simulink model "q_heli_2d_ff_lqr_i_no_joystick"  (Simulink 8.8)
settings: Solver=FixedStepAuto  StartTime=0.0  StopTime=inf  FixedStep=1e-3  MaxStep=10  RelTol=1e-3  AbsTol=1e-3
values from neighbouring files (symbols this model uses):
  B_p = 0.3    [parametri.m]
  B_y = 0.45    [parametri.m]
  g = 9.81    [parametri.m]    (also in setup_heli_2d_configuration.m)
  J_eq_p = J_p - m_heli*l_cm^2    (= 0.014688525)    [parametri.m]    (also in setup_heli_2d_configuration.m = 0.0181734333333)
  J_eq_y = J_y - m_heli*l_cm^2    (= 0.016488525)    [parametri.m]    (also in setup_heli_2d_configuration.m = 0.02311385)
  K_AMP = 1    [setup_lab_heli_2d.m]
  K_EC_P = 2 * pi / 2400    (= 0.00261799387799)    [setup_lab_heli_2d.m]
  K_EC_Y = 2 * pi / 2400    (= 0.00261799387799)    [setup_lab_heli_2d.m]
  K_ff = 1    [setup_lab_heli_2d.m]
  K_pp = 0.35 * d_p    (= 0.06825)    [parametri.m]    (also in setup_heli_2d_configuration.m = 0.18)
  K_py = 0.018    [parametri.m]    (also in setup_heli_2d_configuration.m = 0.06875)
  K_yp = 0.018    [parametri.m]    (also in setup_heli_2d_configuration.m = 0.06875)
  K_yy = 0.35 * d_y    (= 0.06475)    [parametri.m]    (also in setup_heli_2d_configuration.m = 0.162)
  l_cm = 0.005    [parametri.m]    (also in setup_heli_2d_configuration.m = 0.19)
  m_heli = 2*(m_propeler + m_motor + m_motor_drzac) + m_sipka + m_drzac    (= 0.459)    [parametri.m]    (also in setup_heli_2d_configuration.m = 0.6)
  SAT_INT_ERR_PITCH = 3.2    [setup_lab_heli_2d.m]
  SAT_INT_ERR_YAW = 3.2    [setup_lab_heli_2d.m]
  theta_0 = -47*pi/180    (= -0.820304748437)    [setup_lab_heli_2d.m]
  Tr_p = 1    [setup_lab_heli_2d.m]
  Tr_y = 1    [setup_lab_heli_2d.m]
  VMAX_AMP_P = 3.2    [setup_lab_heli_2d.m]
  VMAX_AMP_Y = 3.2    [setup_lab_heli_2d.m]
  wcf = 2 * pi * 20    (= 125.663706144)    [setup_lab_heli_2d.m]
  zetaf = 0.85    [setup_lab_heli_2d.m]
undefined symbols (not defined in the file or in its folder): K, Ki, MultiQ, PCI, Quanser
libraries: simulink x9, simulink_extras x5, sldrtlib x4
settings Model: Creator=MLevis  LastModifiedBy=Labos1  SimulationMode=external  ExtModeTrigDuration=50000
settings SolverCC: PositivePriorityOrder=on
settings DataIOCC: LimitDataPoints=off  SaveOutput=off  SaveTime=off  SignalLoggingName=sigsOut
settings OptimizationCC: BlockReduction=off  BooleanDataType=off  OptimizeBlockIOStorage=off  BufferReuse=off  GlobalBufferReuse=off  ExpressionFolding=off  ExpressionDepthLimit=2147483647  LocalBlockOutputs=off  InitFltsAndDblsToZero=on  LifeSpan=auto
settings DebuggingCC: SaveWithParameterizedLinksMsg=none  SignalResolutionControl=TryResolveAllWithWarning  MultiTaskDSMMsg=warning  MultiTaskCondExecSysMsg=none
settings HardwareCC: ProdBitPerPointer=64  ProdBitPerSizeT=64  ProdBitPerPtrDiffT=64  ProdLargestAtomicFloat=Float  ProdIntDivRoundTo=Zero  ProdEndianess=LittleEndian  ProdWordSize=64  ProdHWDeviceType=Intel->x86-64 (Windows64)
settings RTWCC: SystemTargetFile=sldrt.tlc  TemplateMakefile=sldrt.tmf  Description=Simulink Desktop Real-Time  RTWCompilerOptimization=on
settings CodeAppCC: MaxIdLength=95
settings SimulinkDesktopRealTimeCC: TargetPreCompLibLocation=C:\Program Files\MATLAB\R2016b\toolbox\sldrt\lib\win64  TargetLangStandard=C89/C90 (ANSI)  SupportVariableSizeSignals=off

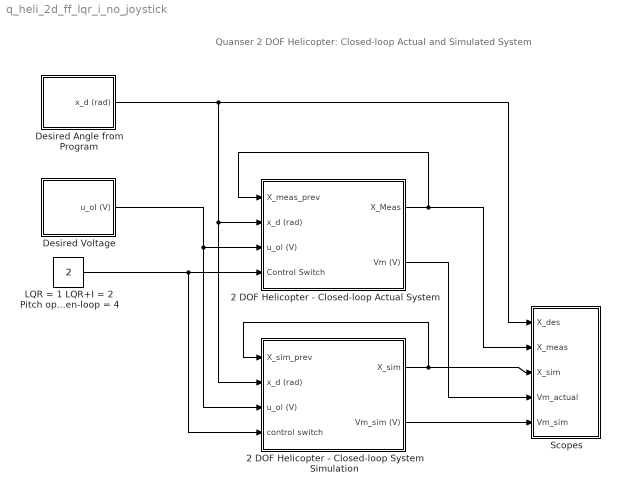
== system q_heli_2d_ff_lqr_i_no_joystick ==
  note: Quanser 2 DOF Helicopter:
      | Closed-loop Actual and Simulated System
  2 DOF Helicopter - Closed-loop Actual System : Subsystem
  2 DOF Helicopter - Closed-loop System Simulation : Subsystem
  Desired Angle from Program : Subsystem
  Desired Voltage : Subsystem
  LQR = 1 LQR+I = 2 Pitch open-loop  = 3 Yaw open-loop = 4 : Constant  Value=2
  Scopes : Subsystem
  wires:
  2 DOF Helicopter - Closed-loop System Simulation/1(X_sim) -> Scopes/3(X_sim), 2 DOF Helicopter - Closed-loop System Simulation/1(X_sim_prev)
  2 DOF Helicopter - Closed-loop Actual System/1(X_Meas) -> 2 DOF Helicopter - Closed-loop Actual System/1(X_meas_prev), Scopes/2(X_meas)
  2 DOF Helicopter - Closed-loop Actual System/2(Vm (V)) -> Scopes/4(Vm_actual)
  LQR = 1 LQR+I = 2 Pitch open-loop  = 3 Yaw open-loop = 4/1 -> 2 DOF Helicopter - Closed-loop Actual System/4(Control Switch), 2 DOF Helicopter - Closed-loop System Simulation/4(control switch)
  2 DOF Helicopter - Closed-loop System Simulation/2(Vm_sim (V)) -> Scopes/5(Vm_sim)
  Desired Voltage/1(u_ol (V)) -> 2 DOF Helicopter - Closed-loop Actual System/3(u_ol (V)), 2 DOF Helicopter - Closed-loop System Simulation/3(u_ol (V))
  Desired Angle from Program/1(x_d (rad)) -> Scopes/1(X_des), 2 DOF Helicopter - Closed-loop Actual System/2(x_d (rad)), 2 DOF Helicopter - Closed-loop System Simulation/2(x_d (rad))

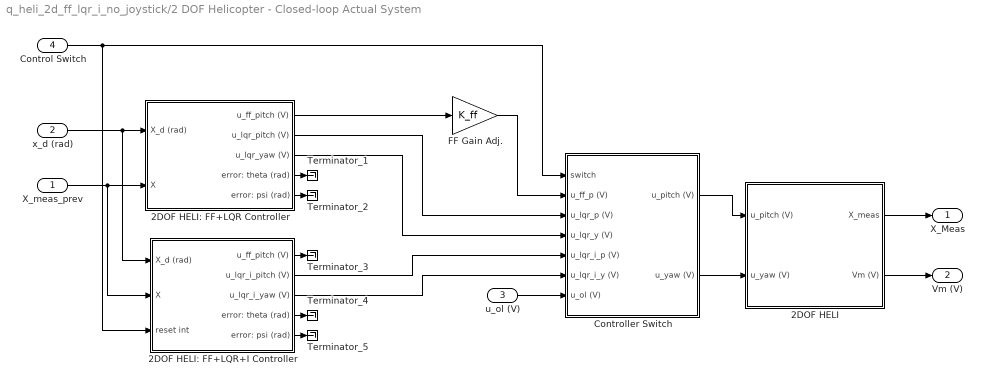
== system q_heli_2d_ff_lqr_i_no_joystick/2 DOF Helicopter - Closed-loop Actual System ==
  X_meas_prev : Inport
  x_d (rad) : Inport  Port=2
  u_ol (V) : Inport  Port=3
  Control Switch : Inport  Port=4
  2DOF HELI : Subsystem
  2DOF HELI: FF+LQR Controller : Subsystem
  2DOF HELI: FF+LQR+I Controller : Subsystem
  Controller Switch : Subsystem
  FF Gain Adj. : Gain  Gain=K_ff
  Terminator_{1..5} (5 alike) : Terminator
  X_Meas : Outport
  Vm (V) : Outport  Port=2
  wires:
  2DOF HELI/1(X_meas) -> X_Meas/1
  2DOF HELI/2(Vm (V)) -> Vm (V)/1
  Control Switch/1 -> 2DOF HELI: FF+LQR+I Controller/3(reset int), Controller Switch/1(switch)
  2DOF HELI: FF+LQR Controller/1(u_ff_pitch (V)) -> FF Gain Adj./1
  x_d (rad)/1 -> 2DOF HELI: FF+LQR Controller/1(X_d (rad)), 2DOF HELI: FF+LQR+I Controller/1(X_d (rad))
  X_meas_prev/1 -> 2DOF HELI: FF+LQR Controller/2(X), 2DOF HELI: FF+LQR+I Controller/2(X)
  2DOF HELI: FF+LQR Controller/3(u_lqr_yaw (V)) -> Controller Switch/4(u_lqr_y (V))
  FF Gain Adj./1 -> Controller Switch/2(u_ff_p (V))
  2DOF HELI: FF+LQR Controller/2(u_lqr_pitch (V)) -> Controller Switch/3(u_lqr_p (V))
  Controller Switch/1(u_pitch (V)) -> 2DOF HELI/1(u_pitch (V))
  Controller Switch/2(u_yaw (V)) -> 2DOF HELI/2(u_yaw (V))
  2DOF HELI: FF+LQR+I Controller/2(u_lqr_i_pitch (V)) -> Controller Switch/5(u_lqr_i_p (V))
  2DOF HELI: FF+LQR+I Controller/3(u_lqr_i_yaw (V)) -> Controller Switch/6(u_lqr_i_y (V))
  u_ol (V)/1 -> Controller Switch/7(u_ol (V))
  2DOF HELI: FF+LQR Controller/4(error: theta (rad)) -> Terminator_1/1
  2DOF HELI: FF+LQR Controller/5(error: psi (rad)) -> Terminator_2/1
  2DOF HELI: FF+LQR+I Controller/1(u_ff_pitch (V)) -> Terminator_3/1
  2DOF HELI: FF+LQR+I Controller/4(error: theta (rad)) -> Terminator_4/1
  2DOF HELI: FF+LQR+I Controller/5(error: psi (rad)) -> Terminator_5/1

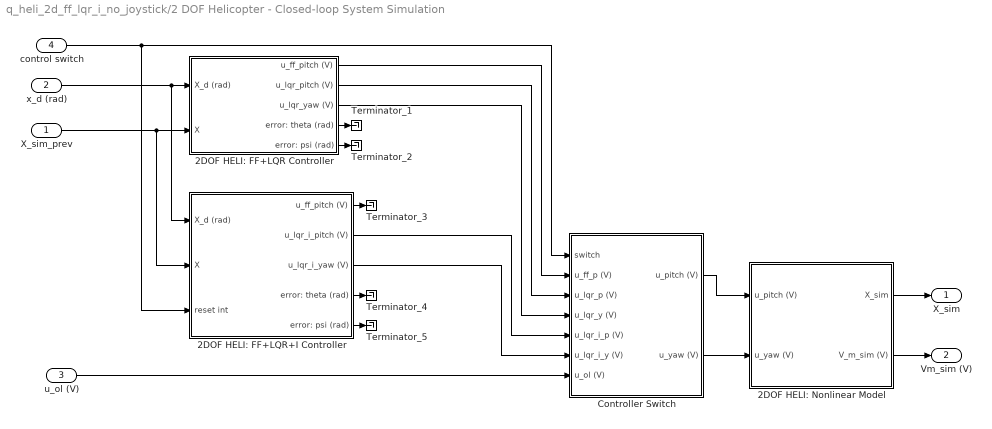
== system q_heli_2d_ff_lqr_i_no_joystick/2 DOF Helicopter - Closed-loop System Simulation ==
  X_sim_prev : Inport
  x_d (rad) : Inport  Port=2
  u_ol (V) : Inport  Port=3
  control switch : Inport  Port=4
  2DOF HELI: FF+LQR Controller : Subsystem
  2DOF HELI: FF+LQR+I Controller : Subsystem
  2DOF HELI: Nonlinear Model : Subsystem
  Controller Switch : Subsystem
  Terminator_{1..5} (5 alike) : Terminator
  X_sim : Outport
  Vm_sim (V) : Outport  Port=2
  wires:
  Controller Switch/2(u_yaw (V)) -> 2DOF HELI: Nonlinear Model/2(u_yaw (V))
  Controller Switch/1(u_pitch (V)) -> 2DOF HELI: Nonlinear Model/1(u_pitch (V))
  x_d (rad)/1 -> 2DOF HELI: FF+LQR+I Controller/1(X_d (rad)), 2DOF HELI: FF+LQR Controller/1(X_d (rad))
  X_sim_prev/1 -> 2DOF HELI: FF+LQR Controller/2(X), 2DOF HELI: FF+LQR+I Controller/2(X)
  2DOF HELI: FF+LQR+I Controller/3(u_lqr_i_yaw (V)) -> Controller Switch/6(u_lqr_i_y (V))
  2DOF HELI: FF+LQR Controller/2(u_lqr_pitch (V)) -> Controller Switch/3(u_lqr_p (V))
  2DOF HELI: FF+LQR Controller/1(u_ff_pitch (V)) -> Controller Switch/2(u_ff_p (V))
  2DOF HELI: FF+LQR Controller/3(u_lqr_yaw (V)) -> Controller Switch/4(u_lqr_y (V))
  2DOF HELI: FF+LQR+I Controller/2(u_lqr_i_pitch (V)) -> Controller Switch/5(u_lqr_i_p (V))
  control switch/1 -> Controller Switch/1(switch), 2DOF HELI: FF+LQR+I Controller/3(reset int)
  2DOF HELI: Nonlinear Model/2(V_m_sim (V)) -> Vm_sim (V)/1
  2DOF HELI: Nonlinear Model/1(X_sim) -> X_sim/1
  u_ol (V)/1 -> Controller Switch/7(u_ol (V))
  2DOF HELI: FF+LQR Controller/4(error: theta (rad)) -> Terminator_1/1
  2DOF HELI: FF+LQR Controller/5(error: psi (rad)) -> Terminator_2/1
  2DOF HELI: FF+LQR+I Controller/1(u_ff_pitch (V)) -> Terminator_3/1
  2DOF HELI: FF+LQR+I Controller/4(error: theta (rad)) -> Terminator_4/1
  2DOF HELI: FF+LQR+I Controller/5(error: psi (rad)) -> Terminator_5/1

== system q_heli_2d_ff_lqr_i_no_joystick/Desired Angle from Program ==
  note: Desired pitch angle
  note: Desired yaw angle
  Amplitude: Pitch (deg) : Gain
  Amplitude: Yaw (deg) : Gain
  Constant : Constant
  Constant: Pitch (deg) : simulink/Math Operations/Slider Gain  low=-50  gain=0  high=25
  Constant: Yaw (deg) : Constant  Value=0
  Mux : Mux  Inputs=2
  Pitch: deg to rad : simulink_extras/Transformations/Degrees to Radians
  Signal Generator: Pitch : SignalGenerator  WaveForm=square  Amplitude=20  Frequency=0.05
  Signal Generator: Yaw : SignalGenerator  WaveForm=square  Amplitude=45  Frequency=0.05
  Sum : Sum  Inputs=|++
  Sum1 : Sum  Inputs=|++
  Yaw: deg to rad : simulink_extras/Transformations/Degrees to Radians
  x_d (rad) : Outport
  wires:
  Pitch: deg to rad/1 -> Mux/1
  Sum/1 -> Pitch: deg to rad/1
  Signal Generator: Pitch/1 -> Amplitude: Pitch (deg)/1
  Amplitude: Pitch (deg)/1 -> Sum/1
  Constant/1 -> Constant: Pitch (deg)/1
  Sum1/1 -> Yaw: deg to rad/1
  Signal Generator: Yaw/1 -> Amplitude: Yaw (deg)/1
  Amplitude: Yaw (deg)/1 -> Sum1/1
  Constant: Yaw (deg)/1 -> Sum1/2
  Mux/1 -> x_d (rad)/1
  Yaw: deg to rad/1 -> Mux/2
  Constant: Pitch (deg)/1 -> Sum/2

== system q_heli_2d_ff_lqr_i_no_joystick/Desired Voltage ==
  note: Desired pitch open-loop voltage
  note: Desired yaw open-loop voltage
  Amplitude: Pitch (V) : Gain  Gain=0
  Amplitude: Yaw (V) : Gain  Gain=0
  Constant: Pitch (V) : Constant  Value=0
  Constant: Yaw (V) : Constant  Value=0
  Mux : Mux  Inputs=2
  Signal Generator: Pitch (V) : SignalGenerator  WaveForm=square  Frequency=0.4
  Signal Generator: Yaw (V) : SignalGenerator  WaveForm=square  Frequency=0.01
  Sum : Sum  Inputs=|++
  Sum1 : Sum  Inputs=|++
  u_ol (V) : Outport
  wires:
  Constant: Pitch (V)/1 -> Sum/2
  Amplitude: Pitch (V)/1 -> Sum/1
  Signal Generator: Pitch (V)/1 -> Amplitude: Pitch (V)/1
  Constant: Yaw (V)/1 -> Sum1/2
  Amplitude: Yaw (V)/1 -> Sum1/1
  Signal Generator: Yaw (V)/1 -> Amplitude: Yaw (V)/1
  Sum/1 -> Mux/1
  Sum1/1 -> Mux/2
  Mux/1 -> u_ol (V)/1

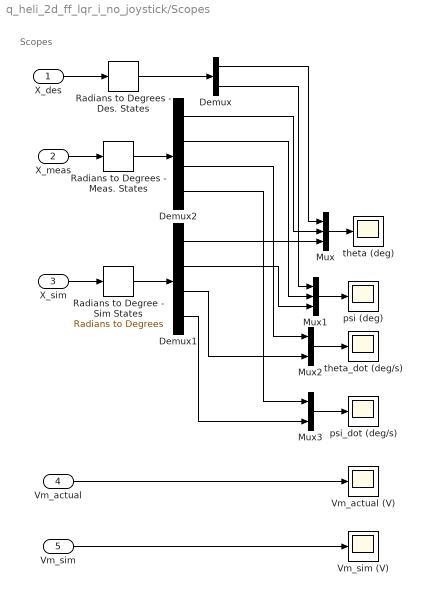
== system q_heli_2d_ff_lqr_i_no_joystick/Scopes ==
  note: Scopes
  X_des : Inport
  X_meas : Inport  Port=2
  X_sim : Inport  Port=3
  Vm_actual : Inport  Port=4
  Vm_sim : Inport  Port=5
  Demux : Demux  Outputs=2
  Demux1 : Demux
  Demux2 : Demux
  Mux : Mux  Inputs=3
  Mux1 : Mux  Inputs=3
  Mux2 : Mux  Inputs=2
  Mux3 : Mux  Inputs=2
  Radians to Degree - Sim States : simulink_extras/Transformations/Radians to Degrees
  Radians to Degrees - Des. States : simulink_extras/Transformations/Radians to Degrees
  Radians to Degrees - Meas. States : simulink_extras/Transformations/Radians to Degrees
  Vm_actual (V) : Scope
  Vm_sim (V) : Scope
  psi (deg) : Scope
  psi_dot (deg/s) : Scope
  theta (deg) : Scope
  theta_dot (deg/s) : Scope
  wires:
  Vm_sim/1 -> Vm_sim (V)/1
  Radians to Degrees - Des. States/1 -> Demux/1
  Demux1/2 -> Mux1/3
  Demux2/2 -> Mux1/2
  Demux/2 -> Mux1/1
  Demux1/1 -> Mux/3
  Demux2/1 -> Mux/2
  Demux/1 -> Mux/1
  X_des/1 -> Radians to Degrees - Des. States/1
  Demux2/3 -> Mux2/1
  Demux2/4 -> Mux3/1
  X_meas/1 -> Radians to Degrees - Meas. States/1
  Radians to Degrees - Meas. States/1 -> Demux2/1
  X_sim/1 -> Radians to Degree - Sim States/1
  Radians to Degree - Sim States/1 -> Demux1/1
  Mux/1 -> theta (deg)/1
  Mux1/1 -> psi (deg)/1
  Mux2/1 -> theta_dot (deg/s)/1
  Mux3/1 -> psi_dot (deg/s)/1
  Demux1/3 -> Mux2/2
  Demux1/4 -> Mux3/2
  Vm_actual/1 -> Vm_actual (V)/1

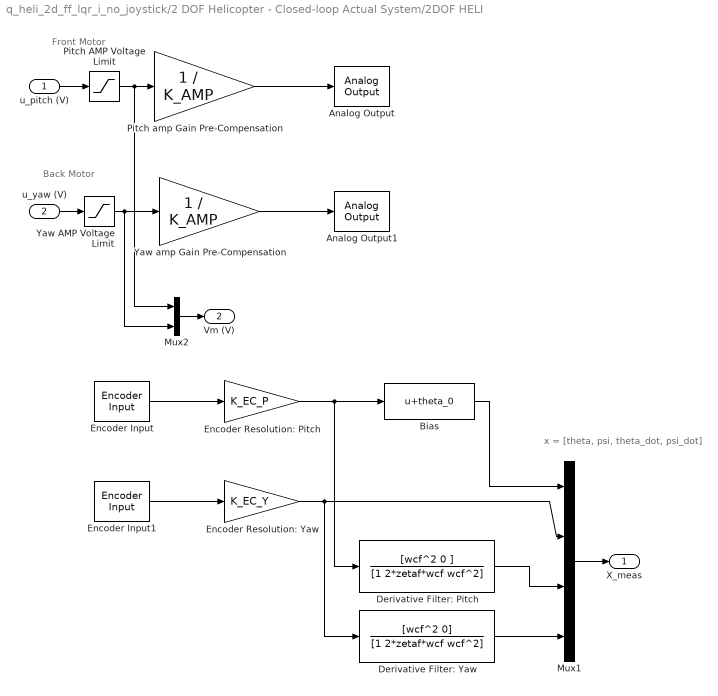
== system q_heli_2d_ff_lqr_i_no_joystick/2 DOF Helicopter - Closed-loop Actual System/2DOF HELI ==
  note: Back Motor
  note: Front Motor
  note: x = [theta, psi, theta_dot, psi_dot]
  u_pitch (V) : Inport
  u_yaw (V) : Inport  Port=2
  Analog Output : sldrtlib/Analog Output  SampleTime=1e-3  MaxMissedTicks=10  ShowMissedTicks=off  YieldWhenWaiting=off  DrvName=Quanser/MultiQ-PCI  DrvAddress=4294967295  DrvOptions=zeros(1,0)  Channels=1  RangeMode=1  VoltRange=1  InitialValue=0  FinalValue=0
      settings: AttributesFormatString=Quanser\nMultiQ-PCI [auto]
  Analog Output1 : sldrtlib/Analog Output  SampleTime=1e-3  MaxMissedTicks=10  ShowMissedTicks=off  YieldWhenWaiting=off  DrvName=Quanser/MultiQ-PCI  DrvAddress=4294967295  DrvOptions=zeros(1,0)  Channels=2  RangeMode=1  VoltRange=1  InitialValue=0  FinalValue=0
      settings: AttributesFormatString=Quanser\nMultiQ-PCI [auto]
  Bias : Bias  Bias=theta_0
  Derivative Filter: Pitch : TransferFcn  Numerator=[wcf^2 0 ]  Denominator=[1 2*zetaf*wcf wcf^2]
  Derivative Filter: Yaw : TransferFcn  Numerator=[wcf^2 0]  Denominator=[1 2*zetaf*wcf wcf^2]
  Encoder Input : sldrtlib/Encoder Input  SampleTime=1e-3  MaxMissedTicks=10  ShowMissedTicks=off  YieldWhenWaiting=off  DrvName=Quanser/MultiQ-PCI  DrvAddress=4294967295  DrvOptions=zeros(1,0)  Channels=1  QuadMode=3  IndexPulse=2  InputFilter=Inf  DataType=1
      settings: AttributesFormatString=Quanser\nMultiQ-PCI [auto]
  Encoder Input1 : sldrtlib/Encoder Input  SampleTime=1e-3  MaxMissedTicks=10  ShowMissedTicks=off  YieldWhenWaiting=off  DrvName=Quanser/MultiQ-PCI  DrvAddress=4294967295  DrvOptions=zeros(1,0)  Channels=2  QuadMode=3  IndexPulse=2  InputFilter=Inf  DataType=1
      settings: AttributesFormatString=Quanser\nMultiQ-PCI [auto]
  "Encoder Resolution: Pitch " : Gain  Gain=K_EC_P
  Encoder Resolution: Yaw : Gain  Gain=K_EC_Y
  Mux1 : Mux
  Mux2 : Mux  Inputs=2
  Pitch AMP Voltage Limit : Saturate  UpperLimit=VMAX_AMP_P  LowerLimit=- VMAX_AMP_P
  Pitch amp Gain Pre-Compensation : Gain  Gain=1 / K_AMP  SaturateOnIntegerOverflow=on  OutDataTypeStr=Inherit: Same as input  ParamDataTypeStr=Inherit: Same as input
  Yaw AMP Voltage Limit : Saturate  UpperLimit=VMAX_AMP_Y  LowerLimit=- VMAX_AMP_Y
  Yaw amp Gain Pre-Compensation : Gain  Gain=1 / K_AMP  SaturateOnIntegerOverflow=on  OutDataTypeStr=Inherit: Same as input  ParamDataTypeStr=Inherit: Same as input
  X_meas : Outport
  Vm (V) : Outport  Port=2
  wires:
  Encoder Resolution: Yaw/1 -> Mux1/2, Derivative Filter: Yaw/1
  Mux2/1 -> Vm (V)/1
  Mux1/1 -> X_meas/1
  u_yaw (V)/1 -> Yaw AMP Voltage Limit/1
  u_pitch (V)/1 -> Pitch AMP Voltage Limit/1
  Yaw AMP Voltage Limit/1 -> Mux2/2, Yaw amp Gain Pre-Compensation/1
  Pitch AMP Voltage Limit/1 -> Mux2/1, Pitch amp Gain Pre-Compensation/1
  Encoder Input/1 -> "Encoder Resolution: Pitch "/1
  "Encoder Resolution: Pitch "/1 -> Bias/1, Derivative Filter: Pitch/1
  Bias/1 -> Mux1/1
  Derivative Filter: Pitch/1 -> Mux1/3
  Derivative Filter: Yaw/1 -> Mux1/4
  Pitch amp Gain Pre-Compensation/1 -> Analog Output/1
  Yaw amp Gain Pre-Compensation/1 -> Analog Output1/1
  Encoder Input1/1 -> Encoder Resolution: Yaw/1

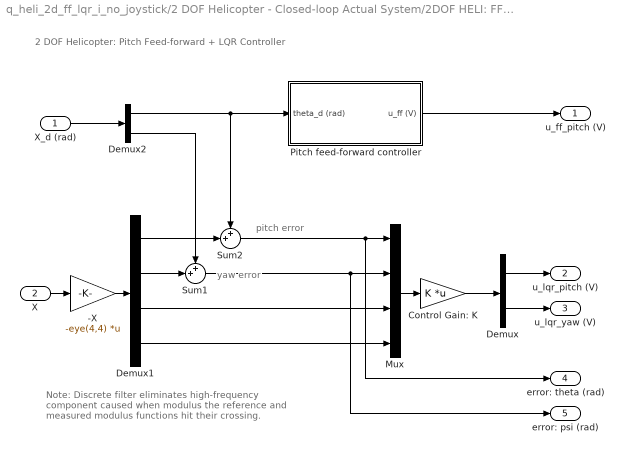
== system q_heli_2d_ff_lqr_i_no_joystick/2 DOF Helicopter - Closed-loop Actual System/2DOF HELI: FF+LQR Controller ==
  note: Note: Discrete filter eliminates high-frequency
      | component caused when modulus the reference
      | and measured modulus functions hit their crossing.
  note: 2 DOF Helicopter:
      | Pitch Feed-forward + LQR Controller
  note: pitch error
  note: yaw error
  X_d (rad) : Inport
  X : Inport  Port=2
  -X : Gain  Gain=-eye(4,4)  Multiplication=Matrix(K*u)
  Control Gain: K : Gain  Gain=K  Multiplication=Matrix(K*u)
  Demux : Demux  Outputs=2
  Demux1 : Demux
  Demux2 : Demux  Outputs=2
  Mux : Mux
  Pitch feed-forward controller : Subsystem
  Sum1 : Sum  Inputs=++|
  Sum2 : Sum  Inputs=++|
  u_ff_pitch (V) : Outport
  u_lqr_pitch (V) : Outport  Port=2
  u_lqr_yaw (V) : Outport  Port=3
  error: theta (rad) : Outport  Port=4
  error: psi (rad) : Outport  Port=5
  wires:
  Sum1/1 -> error: psi (rad)/1, Mux/2
  Demux2/1 -> Sum2/1, Pitch feed-forward controller/1(theta_d (rad))
  Demux2/2 -> Sum1/1
  Demux1/2 -> Sum1/2
  X_d (rad)/1 -> Demux2/1
  Demux1/4 -> Mux/4
  Demux1/3 -> Mux/3
  Mux/1 -> Control Gain: K/1
  Control Gain: K/1 -> Demux/1
  -X/1 -> Demux1/1
  X/1 -> -X/1
  Demux1/1 -> Sum2/2
  Sum2/1 -> error: theta (rad)/1, Mux/1
  Demux/2 -> u_lqr_yaw (V)/1
  Demux/1 -> u_lqr_pitch (V)/1
  Pitch feed-forward controller/1(u_ff (V)) -> u_ff_pitch (V)/1

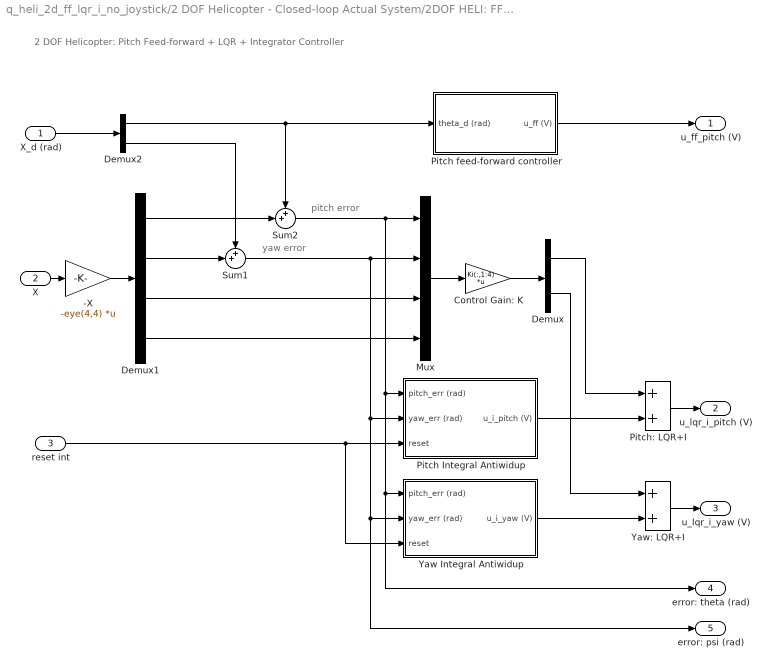
== system q_heli_2d_ff_lqr_i_no_joystick/2 DOF Helicopter - Closed-loop Actual System/2DOF HELI: FF+LQR+I Controller ==
  note: yaw error
  note: pitch error
  note: 2 DOF Helicopter:
      | Pitch Feed-forward + LQR + Integrator Controller
  X_d (rad) : Inport
  X : Inport  Port=2
  reset int : Inport  Port=3
  -X : Gain  Gain=-eye(4,4)  Multiplication=Matrix(K*u)
  Control Gain: K : Gain  Gain=Ki(:,1:4)  Multiplication=Matrix(K*u)
  Demux : Demux  Outputs=2
  Demux1 : Demux
  Demux2 : Demux  Outputs=2
  Mux : Mux
  Pitch Integral Antiwidup : Subsystem
  Pitch feed-forward controller : Subsystem
  Pitch: LQR+I : Sum
  Sum1 : Sum  Inputs=++|
  Sum2 : Sum  Inputs=++|
  Yaw Integral Antiwidup : Subsystem
  Yaw: LQR+I : Sum
  u_ff_pitch (V) : Outport
  u_lqr_i_pitch (V) : Outport  Port=2
  u_lqr_i_yaw (V) : Outport  Port=3
  error: theta (rad) : Outport  Port=4
  error: psi (rad) : Outport  Port=5
  wires:
  reset int/1 -> Pitch Integral Antiwidup/3(reset), Yaw Integral Antiwidup/3(reset)
  Demux1/2 -> Sum1/2
  Demux2/2 -> Sum1/1
  Demux2/1 -> Sum2/1, Pitch feed-forward controller/1(theta_d (rad))
  X_d (rad)/1 -> Demux2/1
  Yaw Integral Antiwidup/1(u_i_yaw (V)) -> Yaw: LQR+I/2
  Demux/2 -> Yaw: LQR+I/1
  Yaw: LQR+I/1 -> u_lqr_i_yaw (V)/1
  Pitch: LQR+I/1 -> u_lqr_i_pitch (V)/1
  Demux/1 -> Pitch: LQR+I/1
  Pitch Integral Antiwidup/1(u_i_pitch (V)) -> Pitch: LQR+I/2
  Pitch feed-forward controller/1(u_ff (V)) -> u_ff_pitch (V)/1
  Sum2/1 -> Mux/1, Yaw Integral Antiwidup/1(pitch_err (rad)), error: theta (rad)/1, Pitch Integral Antiwidup/1(pitch_err (rad))
  Demux1/1 -> Sum2/2
  X/1 -> -X/1
  Sum1/1 -> Yaw Integral Antiwidup/2(yaw_err (rad)), error: psi (rad)/1, Pitch Integral Antiwidup/2(yaw_err (rad)), Mux/2
  -X/1 -> Demux1/1
  Control Gain: K/1 -> Demux/1
  Mux/1 -> Control Gain: K/1
  Demux1/3 -> Mux/3
  Demux1/4 -> Mux/4

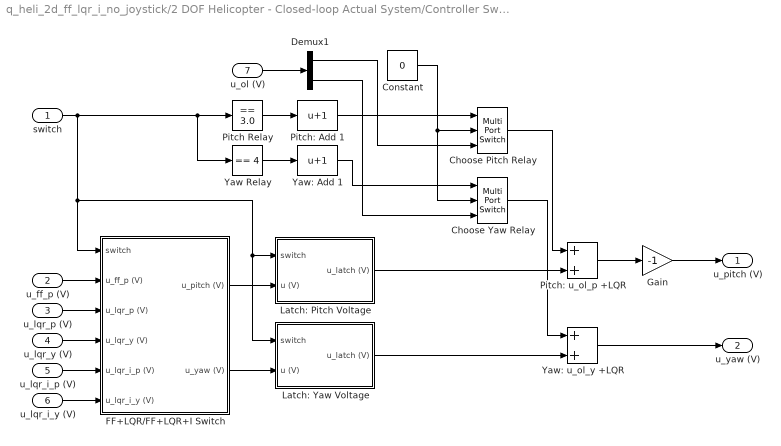
== system q_heli_2d_ff_lqr_i_no_joystick/2 DOF Helicopter - Closed-loop Actual System/Controller Switch ==
  switch : Inport
  u_ff_p (V) : Inport  Port=2
  u_lqr_p (V) : Inport  Port=3
  u_lqr_y (V) : Inport  Port=4
  u_lqr_i_p (V) : Inport  Port=5
  u_lqr_i_y (V) : Inport  Port=6
  u_ol (V) : Inport  Port=7
  Choose Pitch Relay : MultiPortSwitch  Inputs=2
  Choose Yaw Relay : MultiPortSwitch  Inputs=2
  Constant : Constant  Value=0
  Demux1 : Demux  Outputs=2
  FF+LQR/FF+LQR+I Switch : Subsystem
  Gain : Gain  Gain=-1
  Latch: Pitch Voltage : Subsystem
  Latch: Yaw Voltage : Subsystem
  Pitch Relay : simulink/Logic and Bit Operations/Compare To Constant  relop===  const=3.0  OutDataTypeStr=uint8  ZeroCross=off
  Pitch: u_ol_p +LQR : Sum
  Pitch: Add 1 : Bias  Bias=1
  Yaw Relay : simulink/Logic and Bit Operations/Compare To Constant  relop===  const=4  OutDataTypeStr=uint8  ZeroCross=off
  Yaw: u_ol_y +LQR : Sum
  Yaw: Add 1 : Bias  Bias=1
  u_pitch (V) : Outport
  u_yaw (V) : Outport  Port=2
  wires:
  Choose Pitch Relay/1 -> Pitch: u_ol_p +LQR/1
  Choose Yaw Relay/1 -> Yaw: u_ol_y +LQR/1
  Demux1/2 -> Choose Yaw Relay/3
  Demux1/1 -> Choose Pitch Relay/3
  Constant/1 -> Choose Yaw Relay/2, Choose Pitch Relay/2
  Yaw: Add 1/1 -> Choose Yaw Relay/1
  Yaw Relay/1 -> Yaw: Add 1/1
  u_ol (V)/1 -> Demux1/1
  Pitch: Add 1/1 -> Choose Pitch Relay/1
  Pitch Relay/1 -> Pitch: Add 1/1
  Yaw: u_ol_y +LQR/1 -> u_yaw (V)/1
  Pitch: u_ol_p +LQR/1 -> Gain/1
  switch/1 -> Yaw Relay/1, Pitch Relay/1, Latch: Yaw Voltage/1(switch), Latch: Pitch Voltage/1(switch), FF+LQR/FF+LQR+I Switch/1(switch)
  Latch: Yaw Voltage/1(u_latch (V)) -> Yaw: u_ol_y +LQR/2
  Latch: Pitch Voltage/1(u_latch (V)) -> Pitch: u_ol_p +LQR/2
  u_lqr_i_y (V)/1 -> FF+LQR/FF+LQR+I Switch/6(u_lqr_i_y (V))
  u_lqr_i_p (V)/1 -> FF+LQR/FF+LQR+I Switch/5(u_lqr_i_p (V))
  u_lqr_y (V)/1 -> FF+LQR/FF+LQR+I Switch/4(u_lqr_y (V))
  u_lqr_p (V)/1 -> FF+LQR/FF+LQR+I Switch/3(u_lqr_p (V))
  u_ff_p (V)/1 -> FF+LQR/FF+LQR+I Switch/2(u_ff_p (V))
  FF+LQR/FF+LQR+I Switch/2(u_yaw (V)) -> Latch: Yaw Voltage/2(u (V))
  FF+LQR/FF+LQR+I Switch/1(u_pitch (V)) -> Latch: Pitch Voltage/2(u (V))
  Gain/1 -> u_pitch (V)/1

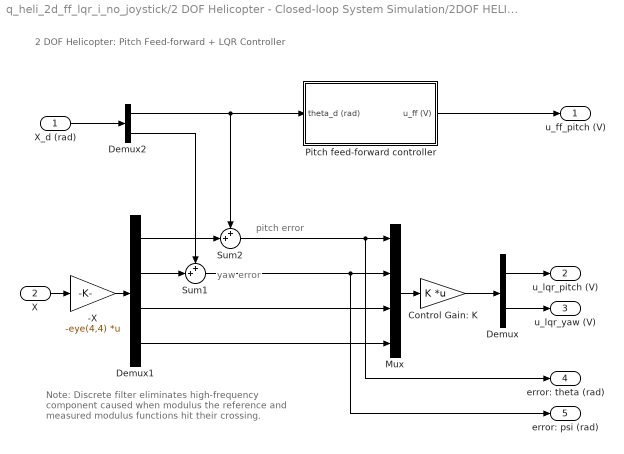
== system q_heli_2d_ff_lqr_i_no_joystick/2 DOF Helicopter - Closed-loop System Simulation/2DOF HELI: FF+LQR Controller ==
  note: Note: Discrete filter eliminates high-frequency
      | component caused when modulus the reference
      | and measured modulus functions hit their crossing.
  note: 2 DOF Helicopter:
      | Pitch Feed-forward + LQR Controller
  note: pitch error
  note: yaw error
  X_d (rad) : Inport
  X : Inport  Port=2
  -X : Gain  Gain=-eye(4,4)  Multiplication=Matrix(K*u)
  Control Gain: K : Gain  Gain=K  Multiplication=Matrix(K*u)
  Demux : Demux  Outputs=2
  Demux1 : Demux
  Demux2 : Demux  Outputs=2
  Mux : Mux
  Pitch feed-forward controller : Subsystem
  Sum1 : Sum  Inputs=++|
  Sum2 : Sum  Inputs=++|
  u_ff_pitch (V) : Outport
  u_lqr_pitch (V) : Outport  Port=2
  u_lqr_yaw (V) : Outport  Port=3
  error: theta (rad) : Outport  Port=4
  error: psi (rad) : Outport  Port=5
  wires:
  Sum1/1 -> error: psi (rad)/1, Mux/2
  Demux2/1 -> Sum2/1, Pitch feed-forward controller/1(theta_d (rad))
  Demux2/2 -> Sum1/1
  Demux1/2 -> Sum1/2
  X_d (rad)/1 -> Demux2/1
  Demux1/4 -> Mux/4
  Demux1/3 -> Mux/3
  Mux/1 -> Control Gain: K/1
  Control Gain: K/1 -> Demux/1
  -X/1 -> Demux1/1
  X/1 -> -X/1
  Demux1/1 -> Sum2/2
  Sum2/1 -> error: theta (rad)/1, Mux/1
  Demux/2 -> u_lqr_yaw (V)/1
  Demux/1 -> u_lqr_pitch (V)/1
  Pitch feed-forward controller/1(u_ff (V)) -> u_ff_pitch (V)/1

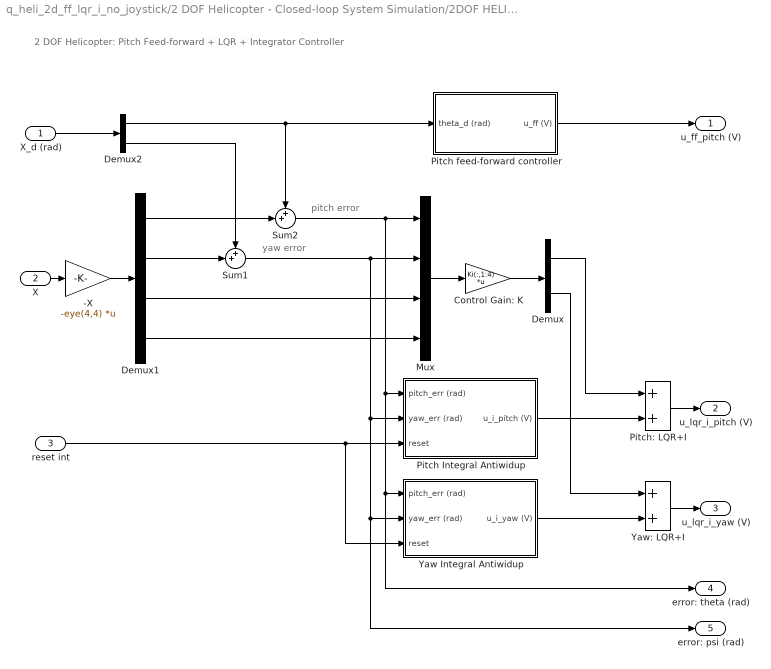
== system q_heli_2d_ff_lqr_i_no_joystick/2 DOF Helicopter - Closed-loop System Simulation/2DOF HELI: FF+LQR+I Controller ==
  note: yaw error
  note: pitch error
  note: 2 DOF Helicopter:
      | Pitch Feed-forward + LQR + Integrator Controller
  X_d (rad) : Inport
  X : Inport  Port=2
  reset int : Inport  Port=3
  -X : Gain  Gain=-eye(4,4)  Multiplication=Matrix(K*u)
  Control Gain: K : Gain  Gain=Ki(:,1:4)  Multiplication=Matrix(K*u)
  Demux : Demux  Outputs=2
  Demux1 : Demux
  Demux2 : Demux  Outputs=2
  Mux : Mux
  Pitch Integral Antiwidup : Subsystem
  Pitch feed-forward controller : Subsystem
  Pitch: LQR+I : Sum
  Sum1 : Sum  Inputs=++|
  Sum2 : Sum  Inputs=++|
  Yaw Integral Antiwidup : Subsystem
  Yaw: LQR+I : Sum
  u_ff_pitch (V) : Outport
  u_lqr_i_pitch (V) : Outport  Port=2
  u_lqr_i_yaw (V) : Outport  Port=3
  error: theta (rad) : Outport  Port=4
  error: psi (rad) : Outport  Port=5
  wires:
  reset int/1 -> Pitch Integral Antiwidup/3(reset), Yaw Integral Antiwidup/3(reset)
  Demux1/2 -> Sum1/2
  Demux2/2 -> Sum1/1
  Demux2/1 -> Sum2/1, Pitch feed-forward controller/1(theta_d (rad))
  X_d (rad)/1 -> Demux2/1
  Yaw Integral Antiwidup/1(u_i_yaw (V)) -> Yaw: LQR+I/2
  Demux/2 -> Yaw: LQR+I/1
  Yaw: LQR+I/1 -> u_lqr_i_yaw (V)/1
  Pitch: LQR+I/1 -> u_lqr_i_pitch (V)/1
  Demux/1 -> Pitch: LQR+I/1
  Pitch Integral Antiwidup/1(u_i_pitch (V)) -> Pitch: LQR+I/2
  Pitch feed-forward controller/1(u_ff (V)) -> u_ff_pitch (V)/1
  Sum2/1 -> Mux/1, Yaw Integral Antiwidup/1(pitch_err (rad)), error: theta (rad)/1, Pitch Integral Antiwidup/1(pitch_err (rad))
  Demux1/1 -> Sum2/2
  X/1 -> -X/1
  Sum1/1 -> Yaw Integral Antiwidup/2(yaw_err (rad)), error: psi (rad)/1, Pitch Integral Antiwidup/2(yaw_err (rad)), Mux/2
  -X/1 -> Demux1/1
  Control Gain: K/1 -> Demux/1
  Mux/1 -> Control Gain: K/1
  Demux1/3 -> Mux/3
  Demux1/4 -> Mux/4

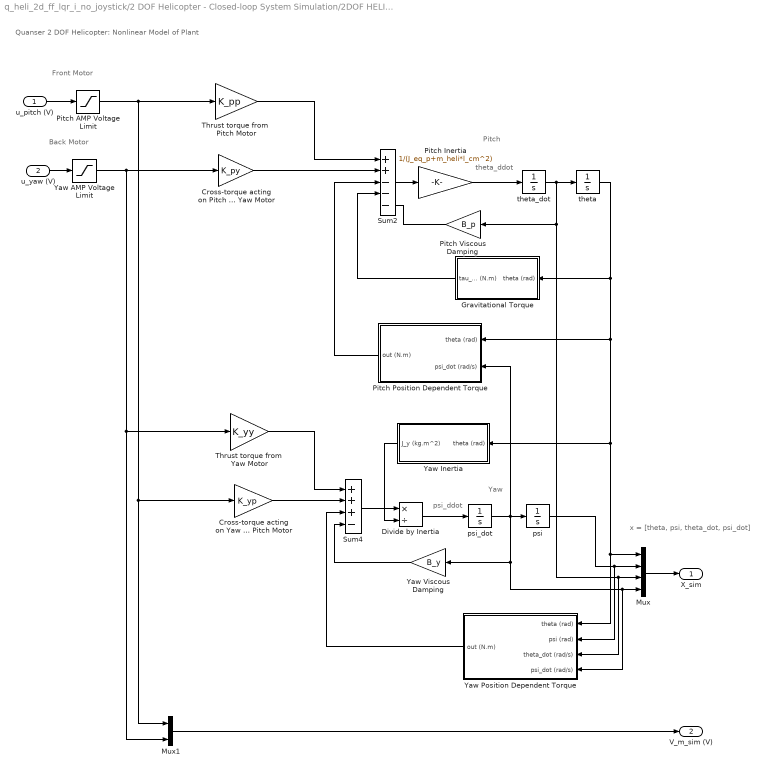
== system q_heli_2d_ff_lqr_i_no_joystick/2 DOF Helicopter - Closed-loop System Simulation/2DOF HELI: Nonlinear Model ==
  note: Back Motor
  note: Front Motor
  note: x = [theta, psi, theta_dot, psi_dot]
  note: Quanser 2 DOF Helicopter: Nonlinear Model of Plant
  note: theta_ddot
  note: psi_ddot
  note: Pitch
  note: Yaw
  u_pitch (V) : Inport
  u_yaw (V) : Inport  Port=2
  Cross-torque acting on Pitch  from Yaw Motor : Gain  Gain=K_py
  Cross-torque acting on Yaw  from Pitch Motor : Gain  Gain=K_yp
  Divide by Inertia : Product  Inputs=*/
  Gravitational Torque : Subsystem
  Mux : Mux
  Mux1 : Mux  Inputs=2
  Pitch AMP Voltage Limit : Saturate  UpperLimit=VMAX_AMP_P  LowerLimit=- VMAX_AMP_P
  Pitch Inertia : Gain  Gain=1/(J_eq_p+m_heli*l_cm^2)
  Pitch Position Dependent Torque : Subsystem
  Pitch Viscous Damping : Gain  Gain=B_p
  Sum2 : Sum  Inputs=++---
  Sum4 : Sum  Inputs=+++-
  Thrust torque from  Pitch Motor : Gain  Gain=K_pp
  Thrust torque from  Yaw Motor : Gain  Gain=K_yy
  Yaw AMP Voltage Limit : Saturate  UpperLimit=VMAX_AMP_Y  LowerLimit=- VMAX_AMP_Y
  Yaw Inertia : Subsystem
  Yaw Position Dependent Torque : Subsystem
  Yaw Viscous Damping : Gain  Gain=B_y
  psi : Integrator
  psi_dot : Integrator
  theta : Integrator  InitialCondition=theta_0  LimitOutput=on  UpperSaturationLimit=-theta_0  LowerSaturationLimit=theta_0
  theta_dot : Integrator
  X_sim : Outport
  V_m_sim (V) : Outport  Port=2
  wires:
  Pitch Position Dependent Torque/1(out (N.m)) -> Sum2/3
  Gravitational Torque/1(tau_g (N.m)) -> Sum2/4
  Pitch Viscous Damping/1 -> Sum2/5
  Cross-torque acting on Pitch  from Yaw Motor/1 -> Sum2/2
  Thrust torque from  Pitch Motor/1 -> Sum2/1
  Yaw Inertia/1(J_y (kg.m^2)) -> Divide by Inertia/2
  Divide by Inertia/1 -> psi_dot/1
  Sum4/1 -> Divide by Inertia/1
  Yaw Position Dependent Torque/1(out (N.m)) -> Sum4/3
  Yaw Viscous Damping/1 -> Sum4/4
  psi/1 -> Yaw Position Dependent Torque/2(psi (rad)), Mux/2
  Mux1/1 -> V_m_sim (V)/1
  Yaw AMP Voltage Limit/1 -> Thrust torque from  Yaw Motor/1, Mux1/2, Cross-torque acting on Pitch  from Yaw Motor/1
  Pitch AMP Voltage Limit/1 -> Mux1/1, Cross-torque acting on Yaw  from Pitch Motor/1, Thrust torque from  Pitch Motor/1
  Mux/1 -> X_sim/1
  theta/1 -> Gravitational Torque/1(theta (rad)), Pitch Position Dependent Torque/1(theta (rad)), Yaw Position Dependent Torque/1(theta (rad)), Mux/1, Yaw Inertia/1(theta (rad))
  Sum2/1 -> Pitch Inertia/1
  Pitch Inertia/1 -> theta_dot/1
  theta_dot/1 -> Pitch Viscous Damping/1, Yaw Position Dependent Torque/3(theta_dot (rad/s)), Mux/3, theta/1
  Thrust torque from  Yaw Motor/1 -> Sum4/1
  Cross-torque acting on Yaw  from Pitch Motor/1 -> Sum4/2
  psi_dot/1 -> Yaw Viscous Damping/1, Yaw Position Dependent Torque/4(psi_dot (rad/s)), Mux/4, Pitch Position Dependent Torque/2(psi_dot (rad/s)), psi/1
  u_pitch (V)/1 -> Pitch AMP Voltage Limit/1
  u_yaw (V)/1 -> Yaw AMP Voltage Limit/1

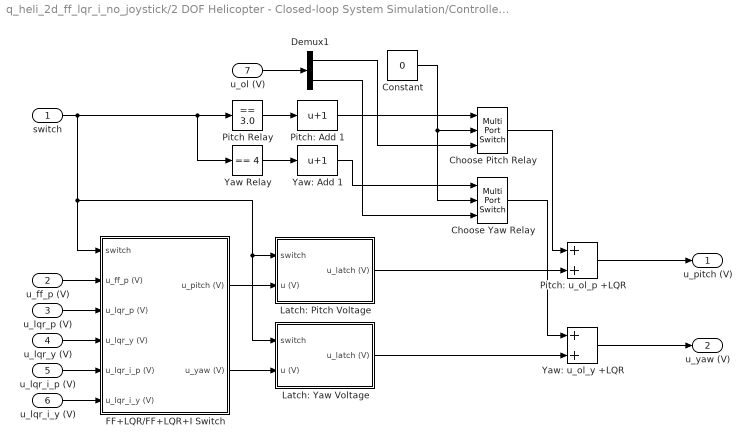
== system q_heli_2d_ff_lqr_i_no_joystick/2 DOF Helicopter - Closed-loop System Simulation/Controller Switch ==
  switch : Inport
  u_ff_p (V) : Inport  Port=2
  u_lqr_p (V) : Inport  Port=3
  u_lqr_y (V) : Inport  Port=4
  u_lqr_i_p (V) : Inport  Port=5
  u_lqr_i_y (V) : Inport  Port=6
  u_ol (V) : Inport  Port=7
  Choose Pitch Relay : MultiPortSwitch  Inputs=2
  Choose Yaw Relay : MultiPortSwitch  Inputs=2
  Constant : Constant  Value=0
  Demux1 : Demux  Outputs=2
  FF+LQR/FF+LQR+I Switch : Subsystem
  Latch: Pitch Voltage : Subsystem
  Latch: Yaw Voltage : Subsystem
  Pitch Relay : simulink/Logic and Bit Operations/Compare To Constant  relop===  const=3.0  OutDataTypeStr=uint8  ZeroCross=off
  Pitch: u_ol_p +LQR : Sum
  Pitch: Add 1 : Bias  Bias=1
  Yaw Relay : simulink/Logic and Bit Operations/Compare To Constant  relop===  const=4  OutDataTypeStr=uint8  ZeroCross=off
  Yaw: u_ol_y +LQR : Sum
  Yaw: Add 1 : Bias  Bias=1
  u_pitch (V) : Outport
  u_yaw (V) : Outport  Port=2
  wires:
  Choose Pitch Relay/1 -> Pitch: u_ol_p +LQR/1
  Choose Yaw Relay/1 -> Yaw: u_ol_y +LQR/1
  Demux1/2 -> Choose Yaw Relay/3
  Demux1/1 -> Choose Pitch Relay/3
  Constant/1 -> Choose Yaw Relay/2, Choose Pitch Relay/2
  Yaw: Add 1/1 -> Choose Yaw Relay/1
  Yaw Relay/1 -> Yaw: Add 1/1
  u_ol (V)/1 -> Demux1/1
  Pitch: Add 1/1 -> Choose Pitch Relay/1
  Pitch Relay/1 -> Pitch: Add 1/1
  Yaw: u_ol_y +LQR/1 -> u_yaw (V)/1
  switch/1 -> Yaw Relay/1, Pitch Relay/1, Latch: Yaw Voltage/1(switch), Latch: Pitch Voltage/1(switch), FF+LQR/FF+LQR+I Switch/1(switch)
  Latch: Yaw Voltage/1(u_latch (V)) -> Yaw: u_ol_y +LQR/2
  Latch: Pitch Voltage/1(u_latch (V)) -> Pitch: u_ol_p +LQR/2
  u_lqr_i_y (V)/1 -> FF+LQR/FF+LQR+I Switch/6(u_lqr_i_y (V))
  u_lqr_i_p (V)/1 -> FF+LQR/FF+LQR+I Switch/5(u_lqr_i_p (V))
  u_lqr_y (V)/1 -> FF+LQR/FF+LQR+I Switch/4(u_lqr_y (V))
  u_lqr_p (V)/1 -> FF+LQR/FF+LQR+I Switch/3(u_lqr_p (V))
  u_ff_p (V)/1 -> FF+LQR/FF+LQR+I Switch/2(u_ff_p (V))
  FF+LQR/FF+LQR+I Switch/2(u_yaw (V)) -> Latch: Yaw Voltage/2(u (V))
  FF+LQR/FF+LQR+I Switch/1(u_pitch (V)) -> Latch: Pitch Voltage/2(u (V))
  Pitch: u_ol_p +LQR/1 -> u_pitch (V)/1

== system q_heli_2d_ff_lqr_i_no_joystick/2 DOF Helicopter - Closed-loop Actual System/2DOF HELI: FF+LQR Controller/Pitch feed-forward controller ==
  note: Desired pitch angle
  theta_d (rad) : Inport
  Feed-forward Pitch Gain : Gain  Gain=l_cm*m_heli*g / K_pp
  Trigonometric Function : Trigonometry  Operator=cos  OutputSignalType=real
  u_ff (V) : Outport
  wires:
  theta_d (rad)/1 -> Trigonometric Function/1
  Feed-forward Pitch Gain/1 -> u_ff (V)/1
  Trigonometric Function/1 -> Feed-forward Pitch Gain/1

== system q_heli_2d_ff_lqr_i_no_joystick/2 DOF Helicopter - Closed-loop Actual System/2DOF HELI: FF+LQR+I Controller/Pitch Integral Antiwidup ==
  note: Pitch: Integral control with anti-windup.
  note: v
  note: u
  pitch_err (rad) : Inport
  yaw_err (rad) : Inport  Port=2
  reset : Inport  Port=3
  Integral Input  (V/s) : Sum
  Integrator : Integrator  ExternalReset=rising
  Pitch Integral Control Gain: K(1,5) : Gain  Gain=Ki(1,5)  Multiplication=Matrix(K*u)
  Pitch Reset Time : Gain  Gain=1/Tr_p
  Saturate : Saturate  UpperLimit=SAT_INT_ERR_PITCH  LowerLimit=-SAT_INT_ERR_PITCH
  Sum : Sum  Inputs=|++
  Yaw Cross-Integral Control Gain: K(1,6) : Gain  Gain=Ki(1,6)  Multiplication=Matrix(K*u)
  u-v : Sum  Inputs=-+
  u_i_pitch (V) : Outport
  wires:
  Integral Input  (V/s)/1 -> Sum/1
  Yaw Cross-Integral Control Gain: K(1,6)/1 -> Integral Input  (V/s)/2
  Pitch Integral Control Gain: K(1,5)/1 -> Integral Input  (V/s)/1
  yaw_err (rad)/1 -> Yaw Cross-Integral Control Gain: K(1,6)/1
  reset/1 -> Integrator/2
  Pitch Reset Time/1 -> Sum/2
  Sum/1 -> Integrator/1
  u-v/1 -> Pitch Reset Time/1
  Saturate/1 -> u-v/2, u_i_pitch (V)/1
  Integrator/1 -> Saturate/1, u-v/1
  pitch_err (rad)/1 -> Pitch Integral Control Gain: K(1,5)/1

== system q_heli_2d_ff_lqr_i_no_joystick/2 DOF Helicopter - Closed-loop Actual System/2DOF HELI: FF+LQR+I Controller/Pitch feed-forward controller ==
  note: Desired pitch angle
  theta_d (rad) : Inport
  Feed-forward Pitch Gain : Gain  Gain=l_cm*m_heli*g / K_pp
  Trigonometric Function : Trigonometry  Operator=cos  OutputSignalType=real
  u_ff (V) : Outport
  wires:
  theta_d (rad)/1 -> Trigonometric Function/1
  Feed-forward Pitch Gain/1 -> u_ff (V)/1
  Trigonometric Function/1 -> Feed-forward Pitch Gain/1

== system q_heli_2d_ff_lqr_i_no_joystick/2 DOF Helicopter - Closed-loop Actual System/2DOF HELI: FF+LQR+I Controller/Yaw Integral Antiwidup ==
  note: Yaw: Integral control with anti-windup.
  note: u
  note: v
  pitch_err (rad) : Inport
  yaw_err (rad) : Inport  Port=2
  reset : Inport  Port=3
  Integral Input  (V/s) : Sum
  Integrator : Integrator  ExternalReset=rising
  Pitch Cross-Integral Control Gain: K(2,5) : Gain  Gain=Ki(2,5)  Multiplication=Matrix(K*u)
  Saturate : Saturate  UpperLimit=SAT_INT_ERR_YAW  LowerLimit=-SAT_INT_ERR_YAW
  Sum : Sum  Inputs=|++
  Yaw Integral Control Gain: K(2,6) : Gain  Gain=Ki(2,6)  Multiplication=Matrix(K*u)
  Yaw Reset Time : Gain  Gain=1/Tr_y
  u-v : Sum  Inputs=-+
  u_i_yaw (V) : Outport
  wires:
  Integral Input  (V/s)/1 -> Sum/1
  Pitch Cross-Integral Control Gain: K(2,5)/1 -> Integral Input  (V/s)/2
  Yaw Integral Control Gain: K(2,6)/1 -> Integral Input  (V/s)/1
  pitch_err (rad)/1 -> Pitch Cross-Integral Control Gain: K(2,5)/1
  reset/1 -> Integrator/2
  yaw_err (rad)/1 -> Yaw Integral Control Gain: K(2,6)/1
  Integrator/1 -> u-v/1, Saturate/1
  Saturate/1 -> u_i_yaw (V)/1, u-v/2
  u-v/1 -> Yaw Reset Time/1
  Sum/1 -> Integrator/1
  Yaw Reset Time/1 -> Sum/2

== system q_heli_2d_ff_lqr_i_no_joystick/2 DOF Helicopter - Closed-loop Actual System/Controller Switch/FF+LQR/FF+LQR+I Switch ==
  note: Add corresponding controllers for the pitch and yaw axes of the 2DOF HELI.
  switch : Inport
  u_ff_p (V) : Inport  Port=2
  u_lqr_p (V) : Inport  Port=3
  u_lqr_y (V) : Inport  Port=4
  u_lqr_i_p (V) : Inport  Port=5
  u_lqr_i_y (V) : Inport  Port=6
  Pitch Control  Switch : MultiPortSwitch  Inputs=2
  Pitch: FF+LQR : Sum
  Yaw Control  Switch : MultiPortSwitch  Inputs=2
  u_pitch (V) : Outport
  u_yaw (V) : Outport  Port=2
  wires:
  switch/1 -> Yaw Control  Switch/1, Pitch Control  Switch/1
  u_lqr_i_y (V)/1 -> Yaw Control  Switch/3
  u_lqr_i_p (V)/1 -> Pitch Control  Switch/3
  Yaw Control  Switch/1 -> u_yaw (V)/1
  u_lqr_y (V)/1 -> Yaw Control  Switch/2
  u_lqr_p (V)/1 -> Pitch Control  Switch/2
  Pitch: FF+LQR/1 -> u_pitch (V)/1
  u_ff_p (V)/1 -> Pitch: FF+LQR/1
  Pitch Control  Switch/1 -> Pitch: FF+LQR/2

== system q_heli_2d_ff_lqr_i_no_joystick/2 DOF Helicopter - Closed-loop Actual System/Controller Switch/Latch: Pitch Voltage ==
  switch : Inport
  u (V) : Inport  Port=2
  Add : Sum
  Compare To Constant : simulink/Logic and Bit Operations/Compare To Constant  relop=>=  const=3.0  OutDataTypeStr=uint8  ZeroCross=off
  Constant : Constant
  Memory : Memory
  Switch : MultiPortSwitch  Inputs=2
  u_latch (V) : Outport
  wires:
  Constant/1 -> Add/2
  Compare To Constant/1 -> Add/1
  switch/1 -> Compare To Constant/1
  u (V)/1 -> Switch/2
  Add/1 -> Switch/1
  Memory/1 -> Switch/3
  Switch/1 -> u_latch (V)/1, Memory/1

== system q_heli_2d_ff_lqr_i_no_joystick/2 DOF Helicopter - Closed-loop Actual System/Controller Switch/Latch: Yaw Voltage ==
  switch : Inport
  u (V) : Inport  Port=2
  Add : Sum
  Compare To Constant : simulink/Logic and Bit Operations/Compare To Constant  relop=>=  const=3.0  OutDataTypeStr=uint8  ZeroCross=off
  Constant : Constant
  Memory : Memory
  Switch : MultiPortSwitch  Inputs=2
  u_latch (V) : Outport
  wires:
  Switch/1 -> Memory/1, u_latch (V)/1
  Memory/1 -> Switch/3
  Add/1 -> Switch/1
  u (V)/1 -> Switch/2
  switch/1 -> Compare To Constant/1
  Compare To Constant/1 -> Add/1
  Constant/1 -> Add/2

== system q_heli_2d_ff_lqr_i_no_joystick/2 DOF Helicopter - Closed-loop System Simulation/2DOF HELI: FF+LQR Controller/Pitch feed-forward controller ==
  note: Desired pitch angle
  theta_d (rad) : Inport
  Feed-forward Pitch Gain : Gain  Gain=l_cm*m_heli*g / K_pp
  Trigonometric Function : Trigonometry  Operator=cos  OutputSignalType=real
  u_ff (V) : Outport
  wires:
  theta_d (rad)/1 -> Trigonometric Function/1
  Feed-forward Pitch Gain/1 -> u_ff (V)/1
  Trigonometric Function/1 -> Feed-forward Pitch Gain/1

== system q_heli_2d_ff_lqr_i_no_joystick/2 DOF Helicopter - Closed-loop System Simulation/2DOF HELI: FF+LQR+I Controller/Pitch Integral Antiwidup ==
  note: Pitch: Integral control with anti-windup.
  note: v
  note: u
  pitch_err (rad) : Inport
  yaw_err (rad) : Inport  Port=2
  reset : Inport  Port=3
  Integral Input  (V/s) : Sum
  Integrator : Integrator  ExternalReset=rising
  Pitch Integral Control Gain: K(1,5) : Gain  Gain=Ki(1,5)  Multiplication=Matrix(K*u)
  Pitch Reset Time : Gain  Gain=1/Tr_p
  Saturate : Saturate  UpperLimit=SAT_INT_ERR_PITCH  LowerLimit=-SAT_INT_ERR_PITCH
  Sum : Sum  Inputs=|++
  Yaw Cross-Integral Control Gain: K(1,6) : Gain  Gain=Ki(1,6)  Multiplication=Matrix(K*u)
  u-v : Sum  Inputs=-+
  u_i_pitch (V) : Outport
  wires:
  Integral Input  (V/s)/1 -> Sum/1
  Yaw Cross-Integral Control Gain: K(1,6)/1 -> Integral Input  (V/s)/2
  Pitch Integral Control Gain: K(1,5)/1 -> Integral Input  (V/s)/1
  yaw_err (rad)/1 -> Yaw Cross-Integral Control Gain: K(1,6)/1
  reset/1 -> Integrator/2
  Pitch Reset Time/1 -> Sum/2
  Sum/1 -> Integrator/1
  u-v/1 -> Pitch Reset Time/1
  Saturate/1 -> u-v/2, u_i_pitch (V)/1
  Integrator/1 -> Saturate/1, u-v/1
  pitch_err (rad)/1 -> Pitch Integral Control Gain: K(1,5)/1

== system q_heli_2d_ff_lqr_i_no_joystick/2 DOF Helicopter - Closed-loop System Simulation/2DOF HELI: FF+LQR+I Controller/Pitch feed-forward controller ==
  note: Desired pitch angle
  theta_d (rad) : Inport
  Feed-forward Pitch Gain : Gain  Gain=l_cm*m_heli*g / K_pp
  Trigonometric Function : Trigonometry  Operator=cos  OutputSignalType=real
  u_ff (V) : Outport
  wires:
  theta_d (rad)/1 -> Trigonometric Function/1
  Feed-forward Pitch Gain/1 -> u_ff (V)/1
  Trigonometric Function/1 -> Feed-forward Pitch Gain/1

== system q_heli_2d_ff_lqr_i_no_joystick/2 DOF Helicopter - Closed-loop System Simulation/2DOF HELI: FF+LQR+I Controller/Yaw Integral Antiwidup ==
  note: Yaw: Integral control with anti-windup.
  note: u
  note: v
  pitch_err (rad) : Inport
  yaw_err (rad) : Inport  Port=2
  reset : Inport  Port=3
  Integral Input  (V/s) : Sum
  Integrator : Integrator  ExternalReset=rising
  Pitch Cross-Integral Control Gain: K(2,5) : Gain  Gain=Ki(2,5)  Multiplication=Matrix(K*u)
  Saturate : Saturate  UpperLimit=SAT_INT_ERR_YAW  LowerLimit=-SAT_INT_ERR_YAW
  Sum : Sum  Inputs=|++
  Yaw Integral Control Gain: K(2,6) : Gain  Gain=Ki(2,6)  Multiplication=Matrix(K*u)
  Yaw Reset Time : Gain  Gain=1/Tr_y
  u-v : Sum  Inputs=-+
  u_i_yaw (V) : Outport
  wires:
  Integral Input  (V/s)/1 -> Sum/1
  Pitch Cross-Integral Control Gain: K(2,5)/1 -> Integral Input  (V/s)/2
  Yaw Integral Control Gain: K(2,6)/1 -> Integral Input  (V/s)/1
  pitch_err (rad)/1 -> Pitch Cross-Integral Control Gain: K(2,5)/1
  reset/1 -> Integrator/2
  yaw_err (rad)/1 -> Yaw Integral Control Gain: K(2,6)/1
  Integrator/1 -> u-v/1, Saturate/1
  Saturate/1 -> u_i_yaw (V)/1, u-v/2
  u-v/1 -> Yaw Reset Time/1
  Sum/1 -> Integrator/1
  Yaw Reset Time/1 -> Sum/2

== system q_heli_2d_ff_lqr_i_no_joystick/2 DOF Helicopter - Closed-loop System Simulation/2DOF HELI: Nonlinear Model/Gravitational Torque ==
  theta (rad) : Inport
  Trigonometric Function : Trigonometry  Operator=cos  OutputSignalType=real
  m*g*lcm : Gain  Gain=m_heli*g*l_cm
  tau_g (N.m) : Outport
  wires:
  m*g*lcm/1 -> tau_g (N.m)/1
  theta (rad)/1 -> Trigonometric Function/1
  Trigonometric Function/1 -> m*g*lcm/1

== system q_heli_2d_ff_lqr_i_no_joystick/2 DOF Helicopter - Closed-loop System Simulation/2DOF HELI: Nonlinear Model/Pitch Position Dependent Torque ==
  theta (rad) : Inport
  psi_dot (rad/s) : Inport  Port=2
  Product : Product  Inputs=4  RndMeth=Zero
  cos(theta) : Trigonometry  Operator=cos  OutputSignalType=real
  m*lcm^2 : Gain  Gain=m_heli*l_cm^2
  sin(theta) : Trigonometry  OutputSignalType=real
  out (N.m) : Outport
  wires:
  psi_dot (rad/s)/1 -> Product/4, Product/3
  theta (rad)/1 -> cos(theta)/1, sin(theta)/1
  Product/1 -> m*lcm^2/1
  sin(theta)/1 -> Product/1
  cos(theta)/1 -> Product/2
  m*lcm^2/1 -> out (N.m)/1

== system q_heli_2d_ff_lqr_i_no_joystick/2 DOF Helicopter - Closed-loop System Simulation/2DOF HELI: Nonlinear Model/Yaw Inertia ==
  theta (rad) : Inport
  Sum3 : Sum
  Yaw Inertia : Constant  Value=J_eq_y
  cos(theta) : Trigonometry  Operator=cos  OutputSignalType=real
  cos(theta)^2 : Product  RndMeth=Zero
  m_heli*l_cm^2 : Gain  Gain=m_heli*l_cm^2
  J_y (kg.m^2) : Outport
  wires:
  cos(theta)/1 -> cos(theta)^2/2, cos(theta)^2/1
  Sum3/1 -> J_y (kg.m^2)/1
  theta (rad)/1 -> cos(theta)/1
  m_heli*l_cm^2/1 -> Sum3/2
  Yaw Inertia/1 -> Sum3/1
  cos(theta)^2/1 -> m_heli*l_cm^2/1

== system q_heli_2d_ff_lqr_i_no_joystick/2 DOF Helicopter - Closed-loop System Simulation/2DOF HELI: Nonlinear Model/Yaw Position Dependent Torque ==
  theta (rad) : Inport
  psi (rad) : Inport  Port=2
  theta_dot (rad/s) : Inport  Port=3
  psi_dot (rad/s) : Inport  Port=4
  2*m*lcm^2 : Gain  Gain=2*m_heli*l_cm^2
  Product : Product  Inputs=4  RndMeth=Zero
  cos(theta) : Trigonometry  Operator=cos  OutputSignalType=real
  sin(psi) : Trigonometry  OutputSignalType=real
  out (N.m) : Outport
  wires:
  2*m*lcm^2/1 -> out (N.m)/1
  psi_dot (rad/s)/1 -> Product/4
  theta_dot (rad/s)/1 -> Product/3
  sin(psi)/1 -> Product/2
  cos(theta)/1 -> Product/1
  Product/1 -> 2*m*lcm^2/1
  theta (rad)/1 -> cos(theta)/1
  psi (rad)/1 -> sin(psi)/1

== system q_heli_2d_ff_lqr_i_no_joystick/2 DOF Helicopter - Closed-loop System Simulation/Controller Switch/FF+LQR/FF+LQR+I Switch ==
  note: Add corresponding controllers for the pitch and yaw axes of the 2DOF HELI.
  switch : Inport
  u_ff_p (V) : Inport  Port=2
  u_lqr_p (V) : Inport  Port=3
  u_lqr_y (V) : Inport  Port=4
  u_lqr_i_p (V) : Inport  Port=5
  u_lqr_i_y (V) : Inport  Port=6
  Pitch Control  Switch : MultiPortSwitch  Inputs=2
  Pitch: FF+LQR : Sum
  Yaw Control  Switch : MultiPortSwitch  Inputs=2
  u_pitch (V) : Outport
  u_yaw (V) : Outport  Port=2
  wires:
  switch/1 -> Yaw Control  Switch/1, Pitch Control  Switch/1
  u_lqr_i_y (V)/1 -> Yaw Control  Switch/3
  u_lqr_i_p (V)/1 -> Pitch Control  Switch/3
  Yaw Control  Switch/1 -> u_yaw (V)/1
  u_lqr_y (V)/1 -> Yaw Control  Switch/2
  u_lqr_p (V)/1 -> Pitch Control  Switch/2
  u_ff_p (V)/1 -> Pitch: FF+LQR/1
  Pitch Control  Switch/1 -> Pitch: FF+LQR/2
  Pitch: FF+LQR/1 -> u_pitch (V)/1

== system q_heli_2d_ff_lqr_i_no_joystick/2 DOF Helicopter - Closed-loop System Simulation/Controller Switch/Latch: Pitch Voltage ==
  switch : Inport
  u (V) : Inport  Port=2
  Add : Sum
  Compare To Constant : simulink/Logic and Bit Operations/Compare To Constant  relop=>=  const=3.0  OutDataTypeStr=uint8  ZeroCross=off
  Constant : Constant
  Memory : Memory
  Switch : MultiPortSwitch  Inputs=2
  u_latch (V) : Outport
  wires:
  Constant/1 -> Add/2
  Compare To Constant/1 -> Add/1
  switch/1 -> Compare To Constant/1
  u (V)/1 -> Switch/2
  Add/1 -> Switch/1
  Memory/1 -> Switch/3
  Switch/1 -> u_latch (V)/1, Memory/1

== system q_heli_2d_ff_lqr_i_no_joystick/2 DOF Helicopter - Closed-loop System Simulation/Controller Switch/Latch: Yaw Voltage ==
  switch : Inport
  u (V) : Inport  Port=2
  Add : Sum
  Compare To Constant : simulink/Logic and Bit Operations/Compare To Constant  relop=>=  const=3.0  OutDataTypeStr=uint8  ZeroCross=off
  Constant : Constant
  Memory : Memory
  Switch : MultiPortSwitch  Inputs=2
  u_latch (V) : Outport
  wires:
  Switch/1 -> Memory/1, u_latch (V)/1
  Memory/1 -> Switch/3
  Add/1 -> Switch/1
  u (V)/1 -> Switch/2
  switch/1 -> Compare To Constant/1
  Compare To Constant/1 -> Add/1
  Constant/1 -> Add/2
